simulink model "reaction_pendulum_simulink"  (R2021b)
settings: Solver=FixedStepDiscrete  StartTime=0.0  StopTime=inf  FixedStep=h  RelTol=1e-3  EnableMultiTasking=on
PreLoadFcn:
  | warning('off','MATLAB:dispatcher:InexactMatch');
InitFcn:
  | hwinit
values from neighbouring files (symbols this model uses):
  A = [0.989609173212  0  0; 0  1  0.01; -0.000301949872013  -0.0950246262215  0.997224421049]    [MATRICES.mat]    (also in SS_11_5.mat = [0.9904  0  0; 0  1  0.01; -9e-05  -0.033262024  0.99812133]; WEAREGOINGHOMEMATRICES.mat = [0.989609173212  0  0; 0  1  0.01; 0.000423899858033  -0.095; current_SS.mat = [0.989609173212  0  0; 0  1  0.01; -9.34612180115e-05  -0.02; dynamicUpdateModel.m = [1.000494318995348 0.010001647563961 2.391143629140888e-07)
  Aeq = [Aeq; Ax0]    [Manual_MPC_Companion.m]    (also in Manual_MPC_Companion_THURSDAY.m = zeros(n * Np, n_total))
  B = [4.20519003073 0 0]    [MATRICES.mat]    (also in SS_11_5.mat = [4.1334 0 0]; current_SS.mat; dynamicUpdateModel.m = [-1.828407620987413e-04; full_dynamics.m = dsys.B)
  beq = zeros(n_total,1)    [Manual_MPC_Companion.m]    (also in Manual_MPC_Companion_THURSDAY.m = zeros(n * Np, 1))
  C = [1 0 0; 0 1 0]    [MeasModel.m]    (also in SS_11_5.mat = [1  0  0; 0  1  0]; current_SS.mat = [1  0  0; 0  1  0]; full_dynamics.m = dsys.C; full_system_ID.m = sys_est.C)
  h = 0.01    [SS_11_5.mat]    (also in hwinit.m)
  H = diag([kron(ones(1,Np), Q) kron(ones(1,Np), R)])    [Manual_MPC_Companion.m]    (also in Manual_MPC_Companion_THURSDAY.m = blkdiag(Qbar, Rbar))
  lb = [-1e6*ones(nx_total,1); -ones(m*Np,1)]    [Manual_MPC_Companion.m]    (also in Manual_MPC_Companion_THURSDAY.m = [-1e6*ones(nx_total, 1); -ones(nu_total, 1)])
  ub = [1e6*ones(nx_total,1); ones(m*Np,1)]    [Manual_MPC_Companion.m]    (also in Manual_MPC_Companion_THURSDAY.m = [ 1e6*ones(nx_total, 1);  ones(nu_total, 1)])
undefined symbols (not defined in the file or in its folder): cThresh, Discrete, E_ref, g_eff, K, K_bottom, k_e, L, magnitude, Time
libraries: ctrlSharedLib x3, simulink x3, sharedTrackingLibrary x1
settings Model: SimulationMode=external  ExtModeTrigDuration=100000  Creator=user  LastModifiedBy=jackh
settings DataIOCC: SaveFormat=Array  SignalLoggingSaveFormat=ModelDataLogs  SaveOutput=off  SignalLogging=off  DSMLogging=off  SaveTime=off  ReturnWorkspaceOutputs=off
settings OptimizationCC: ExpressionDepthLimit=2147483647  LifeSpan=inf
settings DebuggingCC: UnderspecifiedInitializationDetection=Classic  MergeDetectMultiDrivingBlocksExec=none  SolverPrmCheckMsg=warning  FcnCallInpInsideContextMsg=warning  StateNameClashWarn=warning  SFUnexpectedBacktrackingDiag=warning  SFNoUnconditionalDefaultTransitionDiag=warning  SFExecutionAtInitializationDiag=none  ArithmeticOperatorsInVariantConditions=warning
settings HardwareCC: ProdBitPerPointer=32  ProdBitPerSizeT=32  ProdBitPerPtrDiffT=32  ProdLargestAtomicFloat=None  ProdIntDivRoundTo=Undefined  ProdEndianess=Unspecified  ProdWordSize=32  ProdHWDeviceType=32-bit Generic
settings ModelReferenceCC: PropagateSignalLabelsOutOfModel=off
settings SFSimCC: SimUseLocalCustomCode=off  CustomCodeUndefinedFunction=UseInterfaceOnly
settings RTWCC: Description=rpend RTDAC/USB2 (Visual C/C++)  SystemTargetFile=rtcon_rpend_usb2.tlc  TemplateMakefile=rtcon_rpend_vc_usb2_x64.tmf  RTWUseLocalCustomCode=off
settings CodeAppCC: StateflowObjectComments=on
settings STFCustomTargetCC: ModelReferenceCompliant=off  CombineOutputUpdateFcns=on  MatFileLogging=on  GRTInterface=off  SystemTargetFile=rtcon_rpend_usb2.tlc
settings GRTTargetCC: TargetLangStandard=C89/C90 (ANSI)  ModelReferenceCompliant=off  ParMdlRefBuildCompliant=off  CompOptLevelCompliant=off  ConcurrentExecutionCompliant=off  CPPClassGenCompliant=off  UseToolchainInfoCompliant=off  ExtMode=on  ExtModeMexFile=rtcon_ext_comm
settings ConfigComp: CovMetricSettings=dw  CovSaveCumulativeToWorkspaceVar=on  CovSaveSingleToWorkspaceVar=on  CovExternalEMLEnable=off  CovSFcnEnable=off  CovBoundaryAbsTol=1.0e-5

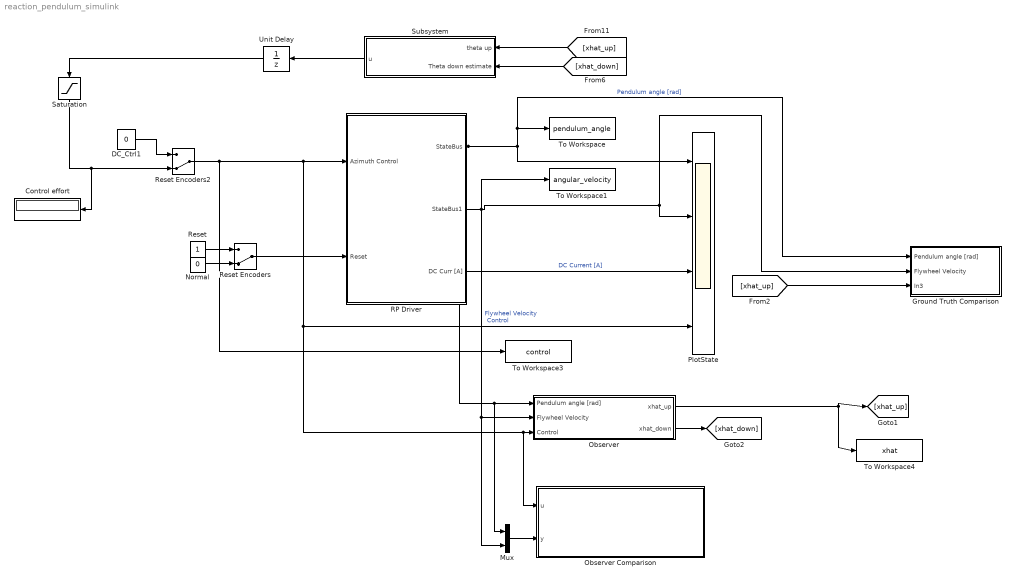
== system reaction_pendulum_simulink ==
  Control effort : Display
  DC_Ctrl1 : Constant  Value=0
  Ground Truth Comparison : Subsystem
  Mux : Mux  Inputs=2
  Normal : Constant  Value=0
  Observer : Subsystem
  Observer Comparison : Subsystem
  PlotState : Scope  NumInputPorts=4
  RP Driver : Subsystem
      mask Display: image(imread('rwp.JPG'))
  Reset : Constant
  Reset Encoders : ManualSwitch  CurrentSetting=0
  Reset Encoders2 : ManualSwitch  CurrentSetting=0
  Saturation : Saturate  UpperLimit=1  LowerLimit=-1
  Subsystem : Subsystem
  To Workspace : ToWorkspace  VariableName=pendulum_angle  SaveFormat=Timeseries  SampleTime=-1
  To Workspace1 : ToWorkspace  VariableName=angular_velocity  SaveFormat=Timeseries  SampleTime=-1
  To Workspace3 : ToWorkspace  VariableName=control  SaveFormat=Timeseries  SampleTime=-1
  To Workspace4 : ToWorkspace  VariableName=xhat  SaveFormat=Timeseries  SampleTime=-1
  Unit Delay : UnitDelay  SampleTime=0.01
  wires:
  Normal/1 -> Reset Encoders/2
  Reset/1 -> Reset Encoders/1
  Reset Encoders/1 -> RP Driver/2(Reset)
  RP Driver/3(DC Curr [A]) -> PlotState/3  "DC Current [A]"
  RP Driver/1(StateBus) -> Ground Truth Comparison/1(Pendulum angle [rad]), To Workspace/1, PlotState/1, Mux/1, Observer/1(Pendulum angle [rad])  "Pendulum angle [rad]"
  Saturation/1 -> Control effort/1, Reset Encoders2/2
  DC_Ctrl1/1 -> Reset Encoders2/1
  Unit Delay/1 -> Saturation/1
  Reset Encoders2/1 -> Observer Comparison/1(u), Observer/3(Control), PlotState/4, RP Driver/1(Azimuth Control), To Workspace3/1  "Control"
  RP Driver/2(StateBus1) -> Mux/2, Observer/2(Flywheel Velocity), Ground Truth Comparison/2(Flywheel Velocity), PlotState/2, To Workspace1/1  "Flywheel Velocity"
  Observer/1(xhat_up) -> [xhat_up], To Workspace4/1
  Observer/2(xhat_down) -> [xhat_down]
  [xhat_up] -> Subsystem/1(theta up)
  [xhat_down] -> Subsystem/2(Theta down estimate)
  Subsystem/1(u) -> Unit Delay/1
  [xhat_up] -> Ground Truth Comparison/3(In3)
  Mux/1 -> Observer Comparison/2(y)

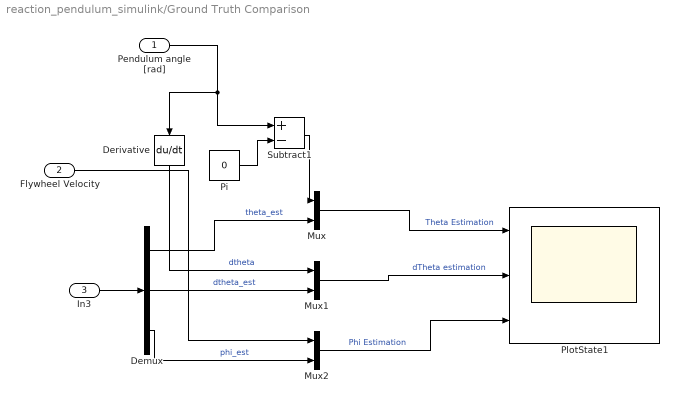
== system reaction_pendulum_simulink/Ground Truth Comparison ==
  Pendulum angle [rad] : Inport
  Flywheel Velocity : Inport  Port=2
  In3 : Inport  Port=3
  Demux : Demux  Outputs=3
  Derivative : Derivative
  Mux : Mux  Inputs=2
  Mux1 : Mux  Inputs=2
  Mux2 : Mux  Inputs=2
  Pi : Constant  Value=0  OutDataTypeStr=Inherit: Inherit via back propagation
  PlotState1 : Scope  NumInputPorts=3
  Subtract1 : Sum  Inputs=+-
  wires:
  Subtract1/1 -> Mux/1
  Mux1/1 -> PlotState1/2  "dTheta estimation"
  Mux/1 -> PlotState1/1  "Theta Estimation"
  Pendulum angle [rad]/1 -> Derivative/1, Subtract1/1
  Demux/1 -> Mux/2  "theta_est"
  Pi/1 -> Subtract1/2
  Demux/2 -> Mux1/2  "dtheta_est"
  Mux2/1 -> PlotState1/3  "Phi Estimation"
  Demux/3 -> Mux2/2  "phi_est"
  Derivative/1 -> Mux1/1  "dtheta"
  Flywheel Velocity/1 -> Mux2/1
  In3/1 -> Demux/1

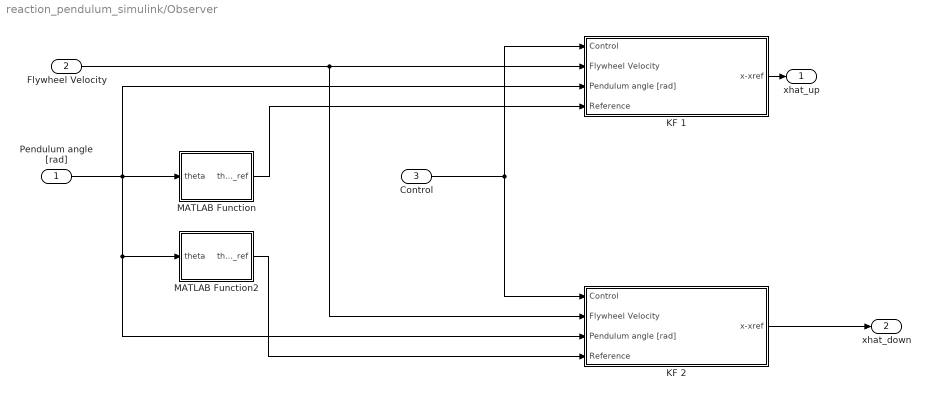
== system reaction_pendulum_simulink/Observer ==
  Pendulum angle [rad] : Inport
  Flywheel Velocity : Inport  Port=2
  Control : Inport  Port=3
  KF 1 : Subsystem
  KF 2 : Subsystem
  MATLAB Function : MATLAB Function  TreatAsAtomicUnit=on
  MATLAB Function2 : MATLAB Function  TreatAsAtomicUnit=on
  xhat_up : Outport
  xhat_down : Outport  Port=2
  wires:
  MATLAB Function2/1(theta_ref) -> KF 2/4(Reference)
  Control/1 -> KF 1/1(Control), KF 2/1(Control)
  MATLAB Function/1(theta_ref) -> KF 1/4(Reference)
  Pendulum angle [rad]/1 -> KF 1/3(Pendulum angle [rad]), KF 2/3(Pendulum angle [rad]), MATLAB Function2/1(theta), MATLAB Function/1(theta)
  Flywheel Velocity/1 -> KF 1/2(Flywheel Velocity), KF 2/2(Flywheel Velocity)
  KF 1/1(x-xref) -> xhat_up/1
  KF 2/1(x-xref) -> xhat_down/1

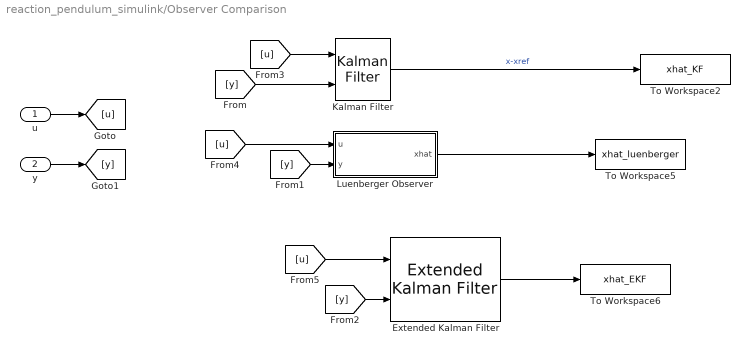
== system reaction_pendulum_simulink/Observer Comparison ==
  u : Inport
  y : Inport  Port=2
  Extended Kalman Filter : sharedTrackingLibrary/Extended Kalman Filter  StateTransitionFcn=dynamicUpdateModel  HasStateTransitionJacobianFcn=off  HasAdditiveProcessNoise=Additive  ProcessNoise=diag([0.00001 0.05 0.0001])  HasTimeVaryingProcessNoise=off  HasStateTransitionFcnExtraArgument=1  InitialState=[0;0;0]  InitialStateCovariance=eye(3)  MeasurementFcn1=measModel  HasMeasurementJacobianFcn1=off  HasMeasurementEnablePort1=off  HasAdditiveMeasurementNoise1=Additive  MeasurementNoise1=diag([0.0001 0.01])  HasTimeVaryingMeasurementNoise1=off  HasMeasurementFcnExtraArgument1=0  HasMeasurementWrapping1=off  MeasurementFcn2=myMeasurementFcn  HasMeasurementJacobianFcn2=off  HasMeasurementEnablePort2=off  HasAdditiveMeasurementNoise2=Additive  MeasurementNoise2=1  HasTimeVaryingMeasurementNoise2=off  HasMeasurementFcnExtraArgument2=0  HasMeasurementWrapping2=off  MeasurementFcn3=myMeasurementFcn  HasMeasurementJacobianFcn3=off  HasMeasurementEnablePort3=off  HasAdditiveMeasurementNoise3=Additive  MeasurementNoise3=1  HasTimeVaryingMeasurementNoise3=off  HasMeasurementFcnExtraArgument3=0  HasMeasurementWrapping3=off  MeasurementFcn4=myMeasurementFcn  HasMeasurementJacobianFcn4=off  HasMeasurementEnablePort4=off  HasAdditiveMeasurementNoise4=Additive  MeasurementNoise4=1  HasTimeVaryingMeasurementNoise4=off  HasMeasurementFcnExtraArgument4=0  HasMeasurementWrapping4=off  MeasurementFcn5=myMeasurementFcn  HasMeasurementJacobianFcn5=off  HasMeasurementEnablePort5=off  HasAdditiveMeasurementNoise5=Additive  MeasurementNoise5=1  HasTimeVaryingMeasurementNoise5=off  HasMeasurementFcnExtraArgument5=0  HasMeasurementWrapping5=off  EnableMultirate=off  StateTransitionFcnSampleTime=1  MeasurementFcn1SampleTime=1  MeasurementFcn2SampleTime=1  MeasurementFcn3SampleTime=1  MeasurementFcn4SampleTime=1  MeasurementFcn5SampleTime=1  UseCurrentEstimator=on  OutputStateCovariance=off  DataType=double  SampleTime=h  NumberOfMeasurements=1
  Kalman Filter : ctrlSharedLib/Kalman Filter  TimeDomain=Discrete-Time  UseCurrentEstimator=on  ModelSource=Individual A, B, C, D matrices  ModelSourceVariable=ss(0.95,1,1,0,1)  A=A  B=B  C=C  D=[0;0]  NumberOfStates=1  NumberOfInputs=1  NumberOfOutputs=1  Ts=-1  InitialEstimateSource=Dialog  X0=0  P0=10  UseK=off  UseGH=off  G=1  TimeInvariantG=on  H=0  TimeInvariantH=on  NumberOfProcessNoiseInputs=1  Q=diag([0.00001 0.05 0.0001])  TimeInvariantQ=on  R=diag([0.0001 0.01])  TimeInvariantR=on  N=0  TimeInvariantN=on  AddInputPort=on  AddEnablePort=off  OutputEstimatedY=off  OutputP=off
  Luenberger Observer : Subsystem
  To Workspace2 : ToWorkspace  VariableName=xhat_KF  SaveFormat=Timeseries  SampleTime=-1
  To Workspace5 : ToWorkspace  VariableName=xhat_luenberger  SaveFormat=Timeseries  SampleTime=-1
  To Workspace6 : ToWorkspace  VariableName=xhat_EKF  SaveFormat=Timeseries  SampleTime=-1
  wires:
  Extended Kalman Filter/1 -> To Workspace6/1
  Kalman Filter/1 -> To Workspace2/1  "x-xref"
  [u] -> Extended Kalman Filter/1
  Luenberger Observer/1(xhat) -> To Workspace5/1
  [y] -> Extended Kalman Filter/2
  [y] -> Luenberger Observer/2(y)
  [u] -> Luenberger Observer/1(u)
  [y] -> Kalman Filter/2
  u/1 -> [u]
  y/1 -> [y]
  [u] -> Kalman Filter/1

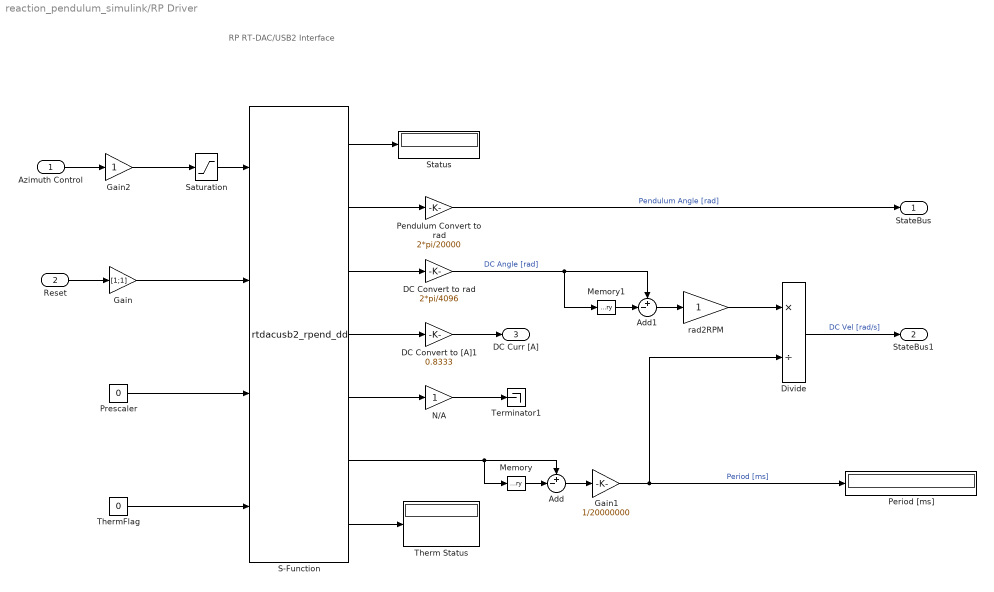
== system reaction_pendulum_simulink/RP Driver ==
  note: RP RT-DAC/USB2
      | Interface
  Azimuth Control : Inport
  Reset : Inport  Port=2
  Add : Sum  Inputs=+-|
  Add1 : Sum  Inputs=+-|
  DC Convert to [A]1 : Gain  Gain=0.8333  SaturateOnIntegerOverflow=on  OutDataTypeStr=Inherit: Same as input  ParamDataTypeStr=Inherit: Same as input
  DC Convert to rad : Gain  Gain=2*pi/4096  SaturateOnIntegerOverflow=on  OutDataTypeStr=Inherit: Same as input  ParamDataTypeStr=Inherit: Same as input
  Divide : Product  Inputs=*/
  Gain : Gain  Gain=[1;1]
  Gain1 : Gain  Gain=1/20000000
  Gain2 : Gain
  Memory : Memory
  Memory1 : Memory
  N/A : Gain  SaturateOnIntegerOverflow=on  OutDataTypeStr=Inherit: Same as input  ParamDataTypeStr=Inherit: Same as input
  Pendulum Convert to rad : Gain  Gain=2*pi/20000  SaturateOnIntegerOverflow=on  OutDataTypeStr=Inherit: Same as input  ParamDataTypeStr=Inherit: Same as input
  Period [ms] : Display
  Prescaler : Constant  Value=0
  S-Function : S-Function  FunctionName=rtdacusb2_rpend_dd  Parameters=1, h  SFunctionDeploymentMode=off  EnableBusSupport=off
  Saturation : Saturate  UpperLimit=1  LowerLimit=-1
  Status : Display
  Terminator1 : Terminator
  Therm Status : Display
  ThermFlag : Constant  Value=0
  rad2RPM : Gain  SaturateOnIntegerOverflow=on  OutDataTypeStr=Inherit: Same as input  ParamDataTypeStr=Inherit: Same as input
  StateBus : Outport  VectorParamsAs1DForOutWhenUnconnected=off
  StateBus1 : Outport  Port=2  VectorParamsAs1DForOutWhenUnconnected=off
  DC Curr [A] : Outport  Port=3  VectorParamsAs1DForOutWhenUnconnected=off
  wires:
  S-Function/7 -> Therm Status/1
  S-Function/5 -> N/A/1
  S-Function/4 -> DC Convert to [A]1/1
  ThermFlag/1 -> S-Function/4
  Prescaler/1 -> S-Function/3
  Gain/1 -> S-Function/2
  DC Convert to [A]1/1 -> DC Curr [A]/1
  Divide/1 -> StateBus1/1  "DC Vel [rad/s]"
  rad2RPM/1 -> Divide/1
  Add1/1 -> rad2RPM/1
  Memory1/1 -> Add1/2
  N/A/1 -> Terminator1/1
  S-Function/6 -> Add/1, Memory/1
  Gain2/1 -> Saturation/1
  Gain1/1 -> Period [ms]/1, Divide/2  "Period [ms]"
  Add/1 -> Gain1/1
  Memory/1 -> Add/2
  DC Convert to rad/1 -> Add1/1, Memory1/1  "DC Angle [rad]"
  S-Function/3 -> DC Convert to rad/1
  Pendulum Convert to rad/1 -> StateBus/1  "Pendulum Angle [rad]"
  S-Function/2 -> Pendulum Convert to rad/1
  S-Function/1 -> Status/1
  Saturation/1 -> S-Function/1
  Reset/1 -> Gain/1
  Azimuth Control/1 -> Gain2/1

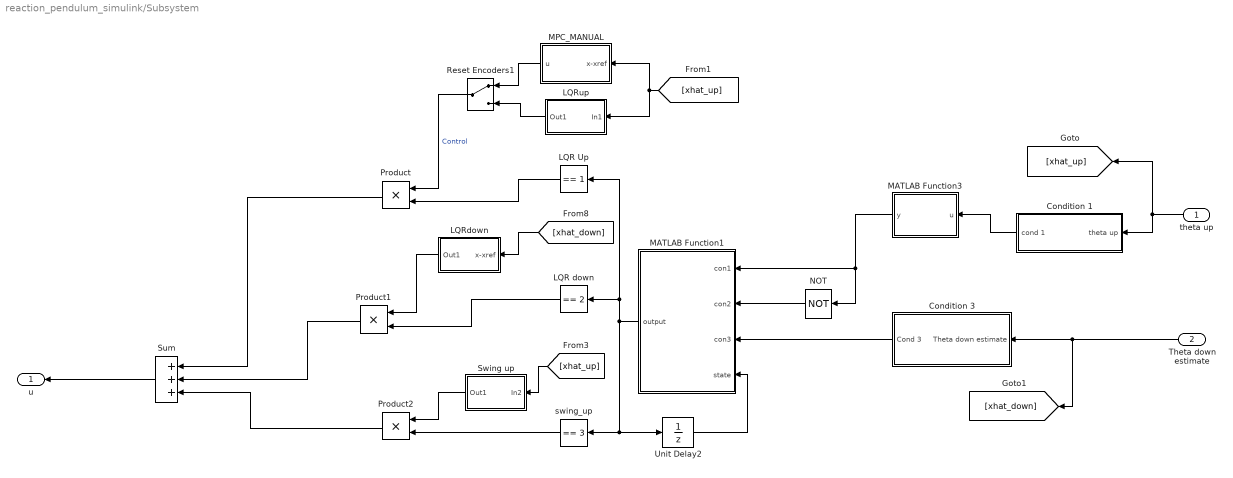
== system reaction_pendulum_simulink/Subsystem ==
  theta up : Inport
  Theta down estimate : Inport  Port=2
  Condition 1 : Subsystem
  Condition 3 : Subsystem
  LQR Up : simulink/Logic and Bit Operations/Compare To Constant  relop===  const=1  OutDataTypeStr=uint8
  LQR down : simulink/Logic and Bit Operations/Compare To Constant  relop===  const=2  OutDataTypeStr=uint8
  LQRdown : Subsystem
  LQRup : Subsystem
  MATLAB Function1 : MATLAB Function  TreatAsAtomicUnit=on
  MATLAB Function3 : MATLAB Function  TreatAsAtomicUnit=on
  MPC_MANUAL : Subsystem
  NOT : Logic  Operator=NOT  IconShape=distinctive  AllPortsSameDT=off  OutDataTypeStr=boolean
  Product : Product
  Product1 : Product
  Product2 : Product
  Reset Encoders1 : ManualSwitch
  Sum : Sum  Inputs=+++
  Swing up : Subsystem
  Unit Delay2 : UnitDelay  InitialCondition=3  SampleTime=h
  swing_up : simulink/Logic and Bit Operations/Compare To Constant  relop===  const=3  OutDataTypeStr=uint8
  u : Outport
  wires:
  NOT/1 -> MATLAB Function1/2(con2)
  [xhat_up] -> Swing up/1(In2)
  [xhat_up] -> MPC_MANUAL/1(x-xref), LQRup/1(In1)
  LQR Up/1 -> Product/2
  MPC_MANUAL/1(u) -> Reset Encoders1/1
  swing_up/1 -> Product2/2
  Product1/1 -> Sum/2
  Product/1 -> Sum/1
  Theta down estimate/1 -> [xhat_down], Condition 3/1(Theta down estimate)
  MATLAB Function1/1(output) -> swing_up/1, Unit Delay2/1, LQR Up/1, LQR down/1
  Unit Delay2/1 -> MATLAB Function1/4(state)
  Reset Encoders1/1 -> Product/1  "Control"
  Condition 1/1(cond 1) -> MATLAB Function3/1(u)
  theta up/1 -> [xhat_up], Condition 1/1(theta up)
  MATLAB Function3/1(y) -> MATLAB Function1/1(con1), NOT/1
  [xhat_down] -> LQRdown/1(x-xref)
  LQR down/1 -> Product1/2
  LQRdown/1(Out1) -> Product1/1
  Swing up/1(Out1) -> Product2/1
  LQRup/1(Out1) -> Reset Encoders1/2
  Condition 3/1(Cond 3) -> MATLAB Function1/3(con3)
  Product2/1 -> Sum/3
  Sum/1 -> u/1

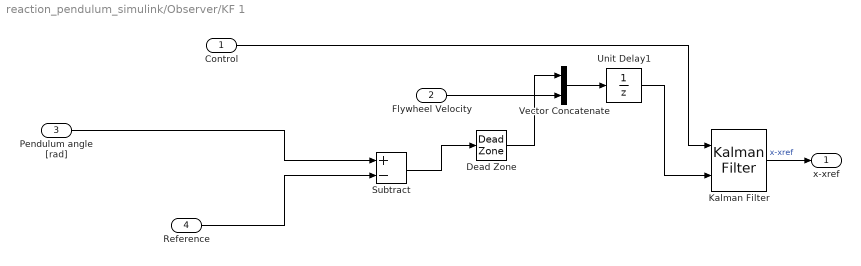
== system reaction_pendulum_simulink/Observer/KF 1 ==
  Control : Inport
  Flywheel Velocity : Inport  Port=2
  Pendulum angle [rad] : Inport  Port=3
  Reference : Inport  Port=4
  Dead Zone : DeadZone  LowerValue=0  UpperValue=0.0  SaturateOnIntegerOverflow=on
  Kalman Filter : ctrlSharedLib/Kalman Filter  TimeDomain=Discrete-Time  UseCurrentEstimator=on  ModelSource=Individual A, B, C, D matrices  ModelSourceVariable=ss(0.95,1,1,0,1)  A=A  B=B  C=C  D=[0;0]  NumberOfStates=1  NumberOfInputs=1  NumberOfOutputs=1  Ts=-1  InitialEstimateSource=Dialog  X0=0  P0=10  UseK=off  UseGH=off  G=1  TimeInvariantG=on  H=0  TimeInvariantH=on  NumberOfProcessNoiseInputs=1  Q=diag([0.00001 0.05 0.0001])  TimeInvariantQ=on  R=diag([0.0001 0.01])  TimeInvariantR=on  N=0  TimeInvariantN=on  AddInputPort=on  AddEnablePort=off  OutputEstimatedY=off  OutputP=off
  Subtract : Sum  Inputs=+-
  Unit Delay1 : UnitDelay  SampleTime=0.01
  Vector Concatenate : Concatenate
  x-xref : Outport
  wires:
  Kalman Filter/1 -> x-xref/1  "x-xref"
  Subtract/1 -> Dead Zone/1
  Reference/1 -> Subtract/2
  Dead Zone/1 -> Vector Concatenate/1
  Flywheel Velocity/1 -> Vector Concatenate/2
  Unit Delay1/1 -> Kalman Filter/2
  Vector Concatenate/1 -> Unit Delay1/1
  Pendulum angle [rad]/1 -> Subtract/1
  Control/1 -> Kalman Filter/1

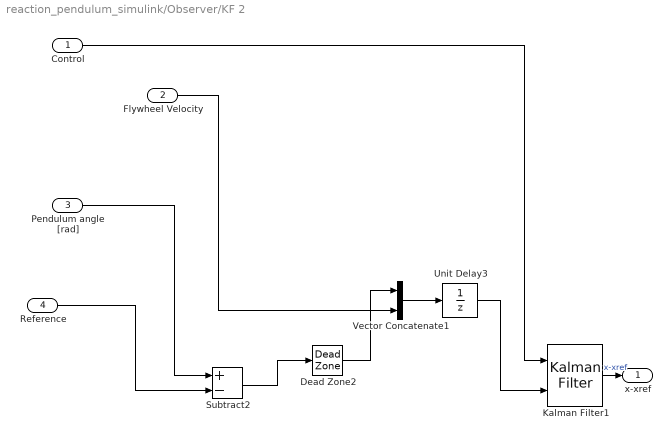
== system reaction_pendulum_simulink/Observer/KF 2 ==
  Control : Inport
  Flywheel Velocity : Inport  Port=2
  Pendulum angle [rad] : Inport  Port=3
  Reference : Inport  Port=4
  Dead Zone2 : DeadZone  LowerValue=0  UpperValue=0.0  SaturateOnIntegerOverflow=on
  Kalman Filter1 : ctrlSharedLib/Kalman Filter  TimeDomain=Discrete-Time  UseCurrentEstimator=on  ModelSource=Individual A, B, C, D matrices  ModelSourceVariable=ss(0.95,1,1,0,1)  A=A  B=B  C=C  D=[0;0]  NumberOfStates=1  NumberOfInputs=1  NumberOfOutputs=1  Ts=-1  InitialEstimateSource=Dialog  X0=0  P0=10  UseK=off  UseGH=off  G=1  TimeInvariantG=on  H=0  TimeInvariantH=on  NumberOfProcessNoiseInputs=1  Q=diag([0.00001 0.05 0.0001])  TimeInvariantQ=on  R=diag([0.0001 0.01])  TimeInvariantR=on  N=0  TimeInvariantN=on  AddInputPort=on  AddEnablePort=off  OutputEstimatedY=off  OutputP=off
  Subtract2 : Sum  Inputs=+-
  Unit Delay3 : UnitDelay  SampleTime=0.01
  Vector Concatenate1 : Concatenate
  x-xref : Outport
  wires:
  Unit Delay3/1 -> Kalman Filter1/2
  Pendulum angle [rad]/1 -> Subtract2/1
  Reference/1 -> Subtract2/2
  Dead Zone2/1 -> Vector Concatenate1/1
  Control/1 -> Kalman Filter1/1
  Subtract2/1 -> Dead Zone2/1
  Vector Concatenate1/1 -> Unit Delay3/1
  Flywheel Velocity/1 -> Vector Concatenate1/2
  Kalman Filter1/1 -> x-xref/1  "x-xref"

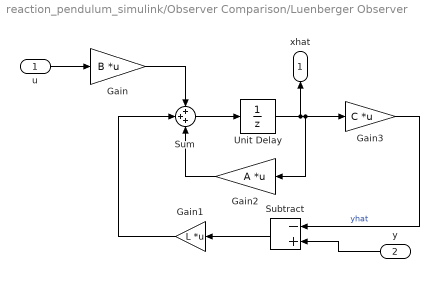
== system reaction_pendulum_simulink/Observer Comparison/Luenberger Observer ==
  u : Inport
  y : Inport  Port=2
  Gain : Gain  Gain=B  Multiplication=Matrix(K*u) (u vector)
  Gain1 : Gain  Gain=L  Multiplication=Matrix(K*u) (u vector)
  Gain2 : Gain  Gain=A  Multiplication=Matrix(K*u) (u vector)
  Gain3 : Gain  Gain=C  Multiplication=Matrix(K*u) (u vector)
  Subtract : Sum  Inputs=-+
  Sum : Sum  Inputs=+++
  Unit Delay : UnitDelay  SampleTime=h
  xhat : Outport
  wires:
  y/1 -> Subtract/2
  Sum/1 -> Unit Delay/1
  Unit Delay/1 -> Gain3/1, Gain2/1, xhat/1
  Gain2/1 -> Sum/3
  u/1 -> Gain/1
  Gain/1 -> Sum/1
  Gain1/1 -> Sum/2
  Gain3/1 -> Subtract/1  "yhat"
  Subtract/1 -> Gain1/1

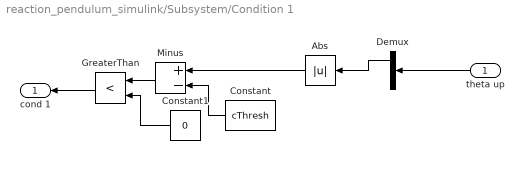
== system reaction_pendulum_simulink/Subsystem/Condition 1 ==
  theta up : Inport
  Abs : Abs
  Constant : Constant  Value=cThresh
  Constant1 : Constant  Value=0
  Demux : Demux  Outputs=3
  GreaterThan : RelationalOperator  Operator=<  OutDataTypeStr=boolean  RndMeth=Simplest
  Minus : Sum  Inputs=+-
  cond 1 : Outport
  wires:
  Constant1/1 -> GreaterThan/2
  theta up/1 -> Demux/1
  Constant/1 -> Minus/2
  Minus/1 -> GreaterThan/1
  GreaterThan/1 -> cond 1/1
  Abs/1 -> Minus/1
  Demux/1 -> Abs/1

== system reaction_pendulum_simulink/Subsystem/Condition 3 ==
  Theta down estimate : Inport
  Abs2 : Abs
  Abs3 : Abs
  Constant2 : Constant  Value=0.1
  Demux3 : Demux  Outputs=3
  GreaterThan1 : RelationalOperator  Operator=<  OutDataTypeStr=boolean  RndMeth=Simplest
  Sum1 : Sum
  Cond 3 : Outport
  wires:
  Demux3/2 -> Abs3/1
  Demux3/1 -> Abs2/1
  Abs2/1 -> Sum1/1
  GreaterThan1/1 -> Cond 3/1
  Constant2/1 -> GreaterThan1/2
  Sum1/1 -> GreaterThan1/1
  Abs3/1 -> Sum1/2
  Theta down estimate/1 -> Demux3/1

== system reaction_pendulum_simulink/Subsystem/LQRdown ==
  x-xref : Inport
  Gain2 : Gain  Gain=-K_bottom  Multiplication=Matrix(K*u) (u vector)
  Out1 : Outport
  wires:
  x-xref/1 -> Gain2/1  "residual (xhat - xref)"
  Gain2/1 -> Out1/1  "u"

== system reaction_pendulum_simulink/Subsystem/LQRup ==
  In1 : Inport
  Gain2 : Gain  Gain=-K  Multiplication=Matrix(K*u) (u vector)
  Out1 : Outport
  wires:
  In1/1 -> Gain2/1  "residual (xhat - xref)"
  Gain2/1 -> Out1/1  "u"

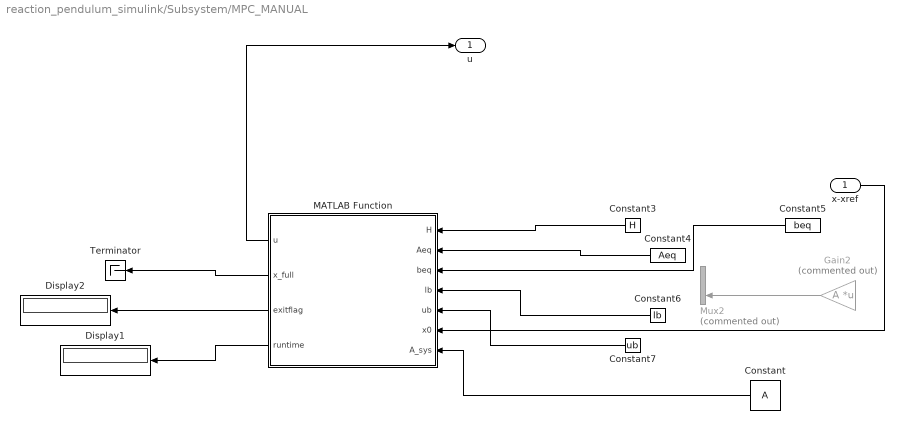
== system reaction_pendulum_simulink/Subsystem/MPC_MANUAL ==
  x-xref : Inport
  Constant : Constant  Value=A  VectorParams1D=off
  Constant3 : Constant  Value=H
  Constant4 : Constant  Value=Aeq
  Constant5 : Constant  Value=beq
  Constant6 : Constant  Value=lb
  Constant7 : Constant  Value=ub
  Display1 : Display
  Display2 : Display
  Gain2 : Gain  Commented=on  Gain=A  Multiplication=Matrix(K*u) (u vector)
  MATLAB Function : MATLAB Function  TreatAsAtomicUnit=on
  Mux2 : Mux  Commented=on  Inputs=2
  Terminator : Terminator
  u : Outport
  wires:
  Constant3/1 -> MATLAB Function/1(H)
  Constant4/1 -> MATLAB Function/2(Aeq)
  Constant5/1 -> MATLAB Function/3(beq)
  Constant6/1 -> MATLAB Function/4(lb)
  MATLAB Function/3(exitflag) -> Display2/1
  Gain2/1 -> Mux2/2
  Constant7/1 -> MATLAB Function/5(ub)
  MATLAB Function/4(runtime) -> Display1/1
  MATLAB Function/2(x_full) -> Terminator/1
  x-xref/1 -> MATLAB Function/6(x0)
  MATLAB Function/1(u) -> u/1
  Constant/1 -> MATLAB Function/7(A_sys)

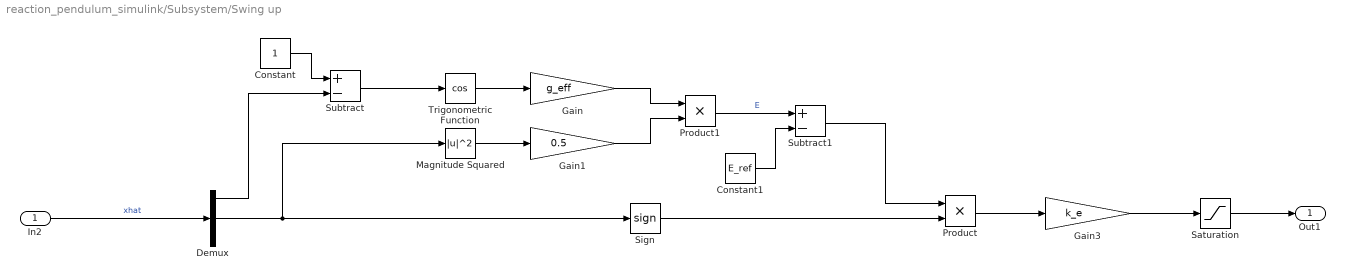
== system reaction_pendulum_simulink/Subsystem/Swing up ==
  In2 : Inport
  Constant : Constant
  Constant1 : Constant  Value=E_ref
  Demux : Demux  Outputs=3
  Gain : Gain  Gain=g_eff
  Gain1 : Gain  Gain=0.5
  Gain3 : Gain  Gain=k_e
  Magnitude Squared : Math  Operator=magnitude^2  SaturateOnIntegerOverflow=on
  Product : Product
  Product1 : Product
  Saturation : Saturate  UpperLimit=0.75  LowerLimit=-0.75
  Sign : Signum
  Subtract : Sum  Inputs=+-
  Subtract1 : Sum  Inputs=+-
  Trigonometric Function : Trigonometry  Operator=cos
  Out1 : Outport
  wires:
  In2/1 -> Demux/1  "xhat"
  Trigonometric Function/1 -> Gain/1
  Magnitude Squared/1 -> Gain1/1
  Gain/1 -> Product1/1
  Gain1/1 -> Product1/2
  Constant/1 -> Subtract/1
  Subtract/1 -> Trigonometric Function/1
  Demux/1 -> Subtract/2
  Sign/1 -> Product/2
  Product1/1 -> Subtract1/1  "E"
  Constant1/1 -> Subtract1/2
  Subtract1/1 -> Product/1
  Product/1 -> Gain3/1
  Gain3/1 -> Saturation/1
  Demux/2 -> Magnitude Squared/1, Sign/1
  Saturation/1 -> Out1/1

== matlab function reaction_pendulum_simulink/Subsystem/MPC_MANUAL/MATLAB Function ==
  data: u output size=1; H input; Aeq input; beq input; lb input; ub input; x_full output; exitflag output; runtime output; x0 input; A_sys input
function [u, x_full, exitflag, runtime] = MPC_short(H, Aeq, beq, lb, ub, x0, A_sys)
tic

n = size(A_sys, 1);
T = size(H, 1) / 4;

% Inject current state into the last n rows of beq
beq(end-n+1 : end) = A_sys * x0;

f      = zeros(size(H, 1), 1);
Aineq  = zeros(0, size(H, 1));
bineq  = zeros(0, 1);
x0_qp  = zeros(size(H, 1), 1);

opts = optimoptions('quadprog', 'Algorithm', 'active-set');

[x_full, ~, exitflag, ~] = quadprog(H, f, Aineq, bineq, Aeq, beq, lb, ub, x0_qp, opts);

u = x_full(3*T + 1);  % first control input u_1
runtime = toc;
end

== matlab function reaction_pendulum_simulink/Observer/MATLAB Function ==
  data: theta input; theta_ref output
function theta_ref = nearestPi(theta)
k = round((theta-pi)/(2*pi));
theta_ref = (2*k + 1)*pi;
end

== matlab function reaction_pendulum_simulink/Subsystem/MATLAB Function1 ==
  data: con1 input; output output; con2 input; con3 input; state input
function output = twswitch(con1, con2, con3, state)
output = 3;
action = 0;
switch state
    case 1
        if con2
            output = 2;
            action = 1;
        end
    case 2
        if con3
            output = 3;
            action = 1;
        end
    case 3
        if con1
            output = 1;
            action = 1;
        end
end
if not(action)
    output = state;
end

== matlab function reaction_pendulum_simulink/Observer/MATLAB Function2 ==
  data: theta input; theta_ref output
function theta_ref = nearest2Pi(theta)
k = round((theta)/(2*pi));
theta_ref = 2*k*pi;
end

== matlab function reaction_pendulum_simulink/Subsystem/MATLAB Function3 ==
  data: u input; y output
function y = delay(u)

N = 3; % 3 consecutive samples

persistent count

if isempty(count)
    count = 0;
end

if u
    count = count + 1;
else
    count = 0;
end

y = count >= N;
